simulink model "Sodel_my_6dof_euler"  (R2017b)
settings: Solver=VariableStepAuto  StartTime=0.0  StopTime=Tsim  RelTol=0.01
values from neighbouring files (symbols this model uses):
  u1max = 25*pi/180    (= 0.436332312999)    [init.m]
  u1min = -25*pi/180    (= -0.436332312999)    [init.m]
  u2max = 10*pi/180    (= 0.174532925199)    [init.m]
  u2min = -25*pi/180    (= -0.436332312999)    [init.m]
  u3max = 30*pi/180    (= 0.523598775598)    [init.m]
  u3min = -30*pi/180    (= -0.523598775598)    [init.m]
  u4max = 10*pi/180    (= 0.174532925199)    [init.m]
  u4min = -0.5*pi/180    (= -0.00872664625997)    [init.m]
  u5max = 10*pi/180    (= 0.174532925199)    [init.m]
  u5min = -0.5*pi/180    (= -0.00872664625997)    [init.m]
  uu = [0; -0.1; 0; 0.0821; 0.0821]    [init.m]
  x0 = [85;0;0;0;0;0;0;0.1;0]    [init.m]
undefined symbols (not defined in the file or in its folder): Earth, sodel_6dof, WGS84
libraries: aerolibfltsims x1, shared6dof x1, aerolibtransform2 x1, dspnetwork x1
settings Model: Creator=Admin  LastModifiedBy=Admin
settings ConfigComp: CovHTMLOptions=-sRT=1 -sVT=0 -aTS=1 -bRG=1 -bTC=1 -hTR=1 -nFC=0 -nFD=1 -scm=1 -bcm=1 -xEv=0 -xEM=0

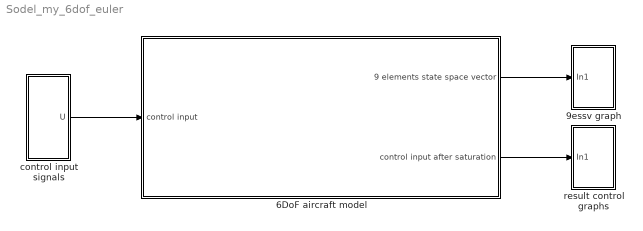
== system Sodel_my_6dof_euler ==
  6DoF aircraft model : Subsystem
  9essv graph : Subsystem
  control input signals : Subsystem
  result control graphs : Subsystem
  wires:
  control input signals/1(U) -> 6DoF aircraft model/1(control input)
  6DoF aircraft model/2(control input after saturation) -> result control graphs/1(In1)
  6DoF aircraft model/1(9 elements state space vector) -> 9essv graph/1(In1)

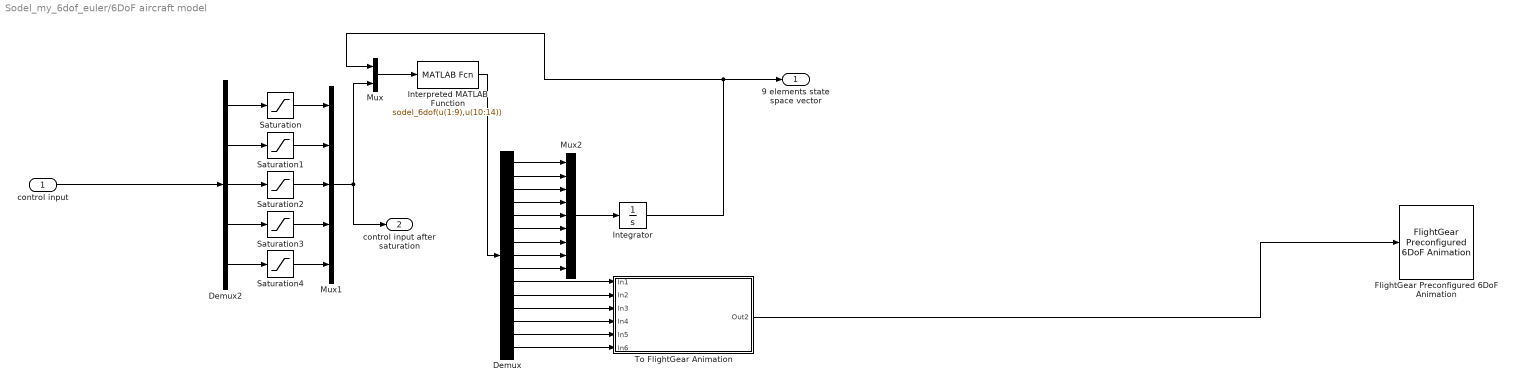
== system Sodel_my_6dof_euler/6DoF aircraft model ==
  control input : Inport
  Demux : Demux  Outputs=15
  Demux2 : Demux  Outputs=5
  FlightGear Preconfigured 6DoF Animation : aerolibfltsims/FlightGear Preconfigured 6DoF Animation  xFlightGearVersion=v2017.1  DestinationIpAddress=127.0.0.1  DestinationPort=5502  SampleTime=1/30
      settings: SourceProductName=Aerospace Blockset
  Integrator : Integrator  InitialCondition=x0
  Interpreted MATLAB Function : MATLABFcn  MATLABFcn=sodel_6dof(u(1:9),u(10:14))
  Mux : Mux  Inputs=2
  Mux1 : Mux  Inputs=5
  Mux2 : Mux  Inputs=9
  Saturation : Saturate  UpperLimit=u1max  LowerLimit=u1min
  Saturation1 : Saturate  UpperLimit=u2max  LowerLimit=u2min
  Saturation2 : Saturate  UpperLimit=u3max  LowerLimit=u3min
  Saturation3 : Saturate  UpperLimit=u4max  LowerLimit=u4min
  Saturation4 : Saturate  UpperLimit=u5max  LowerLimit=u5min
  To FlightGear Animation : Subsystem
  9 elements state space vector : Outport
  control input after saturation : Outport  Port=2
  wires:
  Interpreted MATLAB Function/1 -> Demux/1
  Mux/1 -> Interpreted MATLAB Function/1
  Demux2/2 -> Saturation1/1
  Demux2/4 -> Saturation3/1
  Demux2/5 -> Saturation4/1
  control input/1 -> Demux2/1
  Saturation2/1 -> Mux1/3
  Saturation/1 -> Mux1/1
  Mux1/1 -> Mux/2, control input after saturation/1
  Saturation1/1 -> Mux1/2
  Demux2/3 -> Saturation2/1
  Demux2/1 -> Saturation/1
  Saturation4/1 -> Mux1/5
  Saturation3/1 -> Mux1/4
  Integrator/1 -> Mux/1, 9 elements state space vector/1
  Demux/1 -> Mux2/1
  Demux/2 -> Mux2/2
  Demux/3 -> Mux2/3
  Demux/4 -> Mux2/4
  Demux/5 -> Mux2/5
  Demux/6 -> Mux2/6
  Demux/7 -> Mux2/7
  Demux/8 -> Mux2/8
  Demux/9 -> Mux2/9
  Mux2/1 -> Integrator/1
  Demux/10 -> To FlightGear Animation/1(In1)
  Demux/11 -> To FlightGear Animation/2(In2)
  Demux/12 -> To FlightGear Animation/3(In3)
  Demux/13 -> To FlightGear Animation/4(In4)
  Demux/14 -> To FlightGear Animation/5(In5)
  Demux/15 -> To FlightGear Animation/6(In6)
  To FlightGear Animation/1(Out2) -> FlightGear Preconfigured 6DoF Animation/1

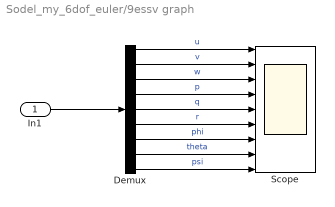
== system Sodel_my_6dof_euler/9essv graph ==
  In1 : Inport
  Demux : Demux  Outputs=9
  Scope : Scope  NumInputPorts=9
  wires:
  In1/1 -> Demux/1
  Demux/1 -> Scope/1  "u"
  Demux/2 -> Scope/2  "v"
  Demux/3 -> Scope/3  "w"
  Demux/5 -> Scope/5  "q"
  Demux/4 -> Scope/4  "p"
  Demux/9 -> Scope/9  "psi"
  Demux/8 -> Scope/8  "theta"
  Demux/6 -> Scope/6  "r"
  Demux/7 -> Scope/7  "phi"

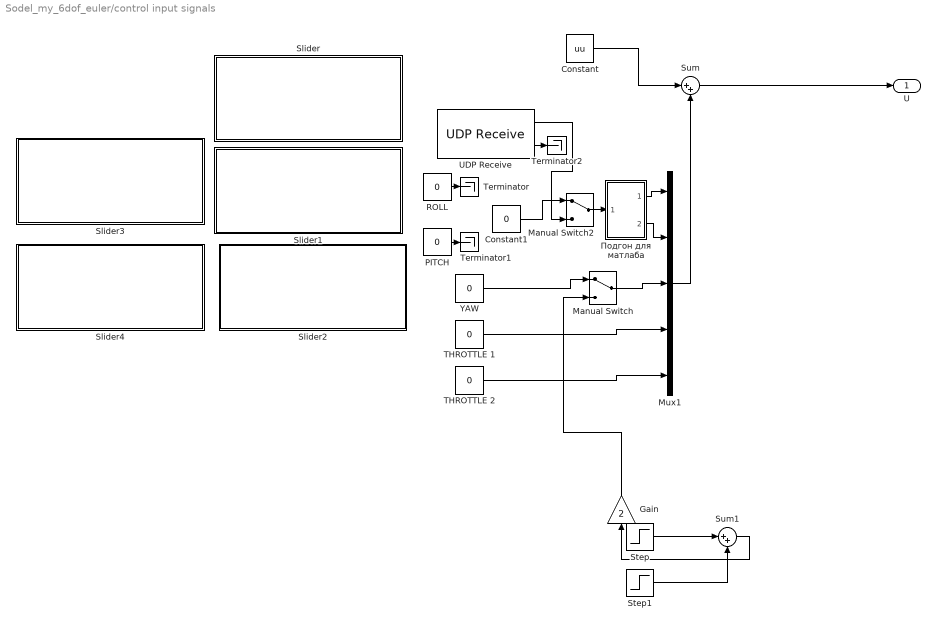
== system Sodel_my_6dof_euler/control input signals ==
  Constant : Constant  Value=uu
  Constant1 : Constant  Value=0
  Gain : Gain  Gain=2
  Manual Switch : ManualSwitch
  Manual Switch2 : ManualSwitch
  Mux1 : Mux  Inputs=5
  PITCH : Constant  Value=0
  "ROLL " : Constant  Value=0
  Slider : Subsystem  DialogController=hmiCreateDDGDialog  IsWebBlock=on  mask(MWDashboardBlock){webBlockId=4142df3a-b1e0-45a1-953a-8fd48c9debc0, webBlockType=slider, ShowInLibBrowser=on, ShowInitialText=on, HMISrcModelName=Sodel_my_6dof_euler}
      mask prompts: webBlockId "WebBlock Id"; webBlockType "WebBlock Type"; HMISrcModelName "Source Model"
      mask help: SimulinkHMI:dialogs:SliderDialogDesc
      mask Help: helpview([docroot '/mapfiles/simulink.map'], 'hmi_slider')
      mask Display:
      | if strcmp(get_param(bdroot(gcb),'BlockDiagramType'), 'library')
      |     image([(matlabroot) '/toolbox/simulink/hmi/icons/Slider.png']);
      | end
  Slider1 : Subsystem  DialogController=hmiCreateDDGDialog  IsWebBlock=on  mask(MWDashboardBlock){webBlockId=67583dfa-0060-4976-b5ff-87e221de8104, webBlockType=slider, ShowInLibBrowser=on, ShowInitialText=on, HMISrcModelName=Sodel_my_6dof_euler}
      mask prompts: webBlockId "WebBlock Id"; webBlockType "WebBlock Type"; HMISrcModelName "Source Model"
      mask help: SimulinkHMI:dialogs:SliderDialogDesc
      mask Help: helpview([docroot '/mapfiles/simulink.map'], 'hmi_slider')
      mask Display:
      | if strcmp(get_param(bdroot(gcb),'BlockDiagramType'), 'library')
      |     image([(matlabroot) '/toolbox/simulink/hmi/icons/Slider.png']);
      | end
  Slider2 : Subsystem  DialogController=hmiCreateDDGDialog  IsWebBlock=on  mask(MWDashboardBlock){webBlockId=c2c1ebfa-c2dd-4ab2-a502-81d1941be81e, webBlockType=slider, ShowInLibBrowser=on, ShowInitialText=on, HMISrcModelName=Sodel_my_6dof_euler}
      mask prompts: webBlockId "WebBlock Id"; webBlockType "WebBlock Type"; HMISrcModelName "Source Model"
      mask help: SimulinkHMI:dialogs:SliderDialogDesc
      mask Help: helpview([docroot '/mapfiles/simulink.map'], 'hmi_slider')
      mask Display:
      | if strcmp(get_param(bdroot(gcb),'BlockDiagramType'), 'library')
      |     image([(matlabroot) '/toolbox/simulink/hmi/icons/Slider.png']);
      | end
  Slider3 : Subsystem  DialogController=hmiCreateDDGDialog  IsWebBlock=on  mask(MWDashboardBlock){webBlockId=440b1d37-215b-4be1-ba7e-1b8ede8ae161, webBlockType=slider, ShowInLibBrowser=on, ShowInitialText=on, HMISrcModelName=Sodel_my_6dof_euler}
      mask prompts: webBlockId "WebBlock Id"; webBlockType "WebBlock Type"; HMISrcModelName "Source Model"
      mask help: SimulinkHMI:dialogs:SliderDialogDesc
      mask Help: helpview([docroot '/mapfiles/simulink.map'], 'hmi_slider')
      mask Display:
      | if strcmp(get_param(bdroot(gcb),'BlockDiagramType'), 'library')
      |     image([(matlabroot) '/toolbox/simulink/hmi/icons/Slider.png']);
      | end
  Slider4 : Subsystem  DialogController=hmiCreateDDGDialog  IsWebBlock=on  mask(MWDashboardBlock){webBlockId=35d14e88-82ea-4b49-8ecc-39665c181e25, webBlockType=slider, ShowInLibBrowser=on, ShowInitialText=on, HMISrcModelName=Sodel_my_6dof_euler}
      mask prompts: webBlockId "WebBlock Id"; webBlockType "WebBlock Type"; HMISrcModelName "Source Model"
      mask help: SimulinkHMI:dialogs:SliderDialogDesc
      mask Help: helpview([docroot '/mapfiles/simulink.map'], 'hmi_slider')
      mask Display:
      | if strcmp(get_param(bdroot(gcb),'BlockDiagramType'), 'library')
      |     image([(matlabroot) '/toolbox/simulink/hmi/icons/Slider.png']);
      | end
  Step : Step  Time=30  After=5*pi/180  SampleTime=0
  Step1 : Step  Time=32  Before=-5*pi/180  After=0  SampleTime=0
  Sum : Sum  Inputs=|++
  Sum1 : Sum  Inputs=|++
  THROTTLE 1 : Constant  Value=0
  THROTTLE 2 : Constant  Value=0
  Terminator : Terminator
  Terminator1 : Terminator
  Terminator2 : Terminator
  UDP Receive : dspnetwork/UDP Receive  localURL='0.0.0.0'  localPort=5005  remoteURL='0.0.0.0'  remotePort=-1  recvBufferSize=16  dims=16  signalDatatype=double  isVarSize=off  showBlockingTime=off  blockingTime=0  sampletime=1  blockPlatform=[]
      settings: SourceProductName=DSP System Toolbox  SourceProductBaseCode=DS
  YAW : Constant  Value=0
  "Подгон для матлаба " : Subsystem
  U : Outport
  wires:
  Mux1/1 -> Sum/2
  Constant/1 -> Sum/1
  THROTTLE 2/1 -> Mux1/5
  Sum/1 -> U/1
  YAW/1 -> Manual Switch/1
  Step/1 -> Sum1/1
  Step1/1 -> Sum1/2
  Sum1/1 -> Gain/1
  Gain/1 -> Manual Switch/2
  THROTTLE 1/1 -> Mux1/4
  Manual Switch/1 -> Mux1/3
  Constant1/1 -> Manual Switch2/1
  UDP Receive/1 -> Manual Switch2/2
  PITCH/1 -> Terminator1/1
  "ROLL "/1 -> Terminator/1
  UDP Receive/2 -> Terminator2/1
  Manual Switch2/1 -> "Подгон для матлаба "/1(In1)
  "Подгон для матлаба "/1(Out1) -> Mux1/1
  "Подгон для матлаба "/2(Out2) -> Mux1/2

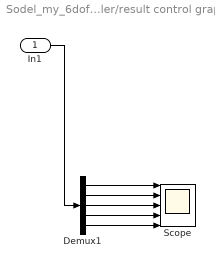
== system Sodel_my_6dof_euler/result control graphs ==
  In1 : Inport
  Demux1 : Demux  Outputs=5
  Scope : Scope  NumInputPorts=5
  wires:
  Demux1/3 -> Scope/3
  Demux1/1 -> Scope/1
  Demux1/4 -> Scope/4
  Demux1/2 -> Scope/2
  Demux1/5 -> Scope/5
  In1/1 -> Demux1/1

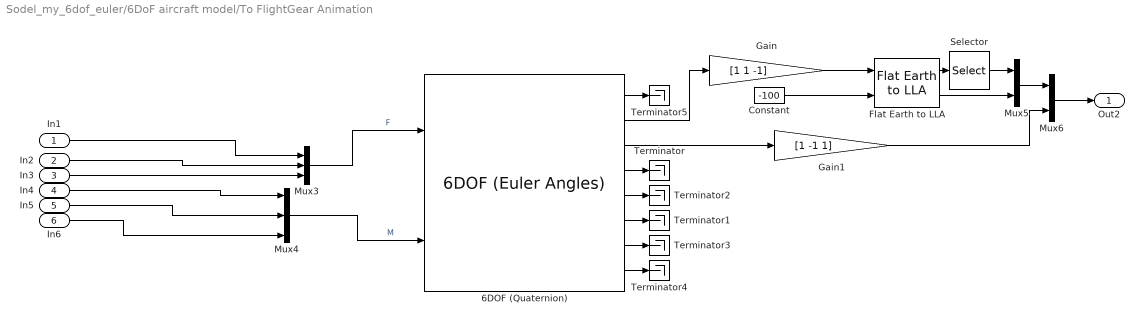
== system Sodel_my_6dof_euler/6DoF aircraft model/To FlightGear Animation ==
  In1 : Inport
  In2 : Inport  Port=2
  In3 : Inport  Port=3
  In4 : Inport  Port=4
  In5 : Inport  Port=5
  In6 : Inport  Port=6
  6DOF (Quaternion) : shared6dof/6DOF (Euler Angles)  units=Metric (MKS)  mtype=Fixed  rep=Quaternion  xme_0=[0 0 0]  Vm_0=[85 0 0]  eul_0=[0 0.1 0]  pm_0=[0 0 0]  mass_0=120000  mass_e=0.5  mass_f=2.0  inertia=|  inertia_e=eye(3)  inertia_f=2*eye(3)  k_quat=1.0  vre_flag=on  abi_flag=off
      | 120000*[40.07 0 -2.0923;
      |         0 64 0;
      |         -2.0923 0 99.92]
      settings: SourceProductBaseCode=AE
  Constant : Constant  Value=-100
  Flat Earth to LLA : aerolibtransform2/Flat Earth to LLA  units=Metric (MKS)  ptype=Earth (WGS84)  F=1/298.257223563  R=6378137  LL0=[37.6272 -122.3896]  psi=0
  Gain : Gain  Gain=[1 1 -1]
  Gain1 : Gain  Gain=[1 -1 1]
  Mux3 : Mux  Inputs=3
  Mux4 : Mux  Inputs=3
  Mux5 : Mux  Inputs=2
  Mux6 : Mux  Inputs=2
  Selector : Selector  IndexMode=Zero-based  InputPortWidth=2  IndexOptions=Index vector (dialog)  Indices=[1 0]  OutputSizes=1
  Terminator{,1..5} (6 alike) : Terminator
  Out2 : Outport
  wires:
  6DOF (Quaternion)/5 -> Terminator2/1
  6DOF (Quaternion)/4 -> Terminator/1
  6DOF (Quaternion)/1 -> Terminator5/1
  6DOF (Quaternion)/8 -> Terminator4/1
  6DOF (Quaternion)/7 -> Terminator3/1
  6DOF (Quaternion)/6 -> Terminator1/1
  In2/1 -> Mux3/2
  In6/1 -> Mux4/3
  In4/1 -> Mux4/1
  In5/1 -> Mux4/2
  In3/1 -> Mux3/3
  Flat Earth to LLA/2 -> Mux5/2
  Flat Earth to LLA/1 -> Selector/1
  Selector/1 -> Mux5/1
  6DOF (Quaternion)/2 -> Gain/1
  Mux5/1 -> Mux6/1
  Constant/1 -> Flat Earth to LLA/2
  6DOF (Quaternion)/3 -> Gain1/1
  In1/1 -> Mux3/1
  Mux4/1 -> 6DOF (Quaternion)/2  "M"
  Mux6/1 -> Out2/1
  Mux3/1 -> 6DOF (Quaternion)/1  "F"
  Gain/1 -> Flat Earth to LLA/1
  Gain1/1 -> Mux6/2

== system Sodel_my_6dof_euler/control input signals/Slider ==

== system Sodel_my_6dof_euler/control input signals/Slider1 ==

== system Sodel_my_6dof_euler/control input signals/Slider2 ==

== system Sodel_my_6dof_euler/control input signals/Slider3 ==

== system Sodel_my_6dof_euler/control input signals/Slider4 ==

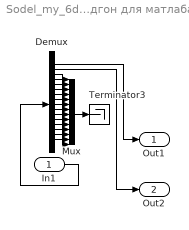
== system Sodel_my_6dof_euler/control input signals/Подгон для матлаба  ==
  In1 : Inport
  Demux : Demux  Outputs=16
  Mux : Mux  Inputs=14
  Terminator3 : Terminator
  Out1 : Outport
  Out2 : Outport  Port=2
  wires:
  In1/1 -> Demux/1
  Demux/1 -> Out1/1
  Demux/3 -> Mux/14
  Mux/1 -> Terminator3/1
  Demux/4 -> Mux/1
  Demux/5 -> Mux/2
  Demux/8 -> Mux/5
  Demux/9 -> Mux/6
  Demux/11 -> Mux/8
  Demux/10 -> Mux/7
  Demux/6 -> Mux/3
  Demux/7 -> Mux/4
  Demux/12 -> Mux/9
  Demux/13 -> Mux/10
  Demux/15 -> Mux/12
  Demux/16 -> Mux/13
  Demux/14 -> Mux/11
  Demux/2 -> Out2/1
